simulink model "model"  (R2024b)
settings: Solver=VariableStepAuto  StartTime=0.0  StopTime=10.0  RelTol=1e-3
undefined symbols (not defined in the file): k
libraries: arduinolib x3, simulink_extras x2, eeGeneralControl x2
settings Model: Creator=eslam  LastModifiedBy=eslam

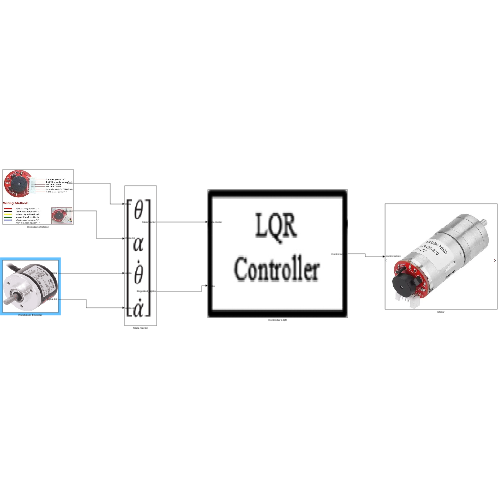
[thumbnail: Simulink's stored preview of the top-level diagram]
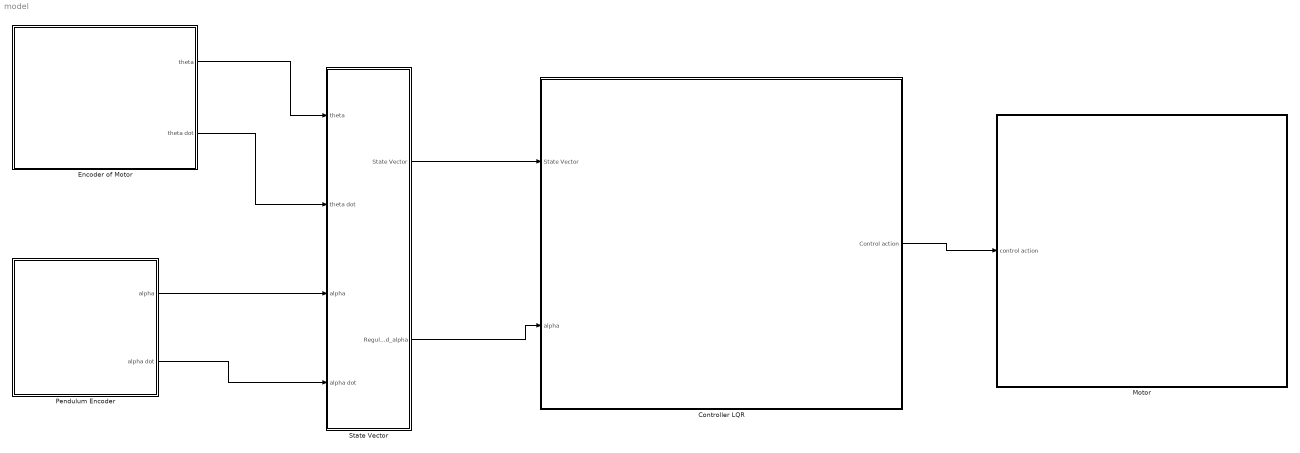
== system model ==
  Controller LQR : Subsystem
      mask Display: image('lqr.PNG');
  Encoder of Motor : Subsystem
      mask Display: image('Motor Encoder.jpeg');
  Motor : Subsystem
      mask Display: image('Motor.png');
  Pendulum Encoder : Subsystem
      mask Display: image('Encoder.png');
  State Vector : Subsystem
      mask Display: image('States.PNG');
  wires:
  Encoder of Motor/1(theta) -> State Vector/1(theta)
  Pendulum Encoder/1(alpha) -> State Vector/3(alpha)
  Encoder of Motor/2(theta dot) -> State Vector/2(theta dot)
  Pendulum Encoder/2(alpha dot) -> State Vector/4(alpha dot)
  State Vector/1(State Vector) -> Controller LQR/1(State Vector)
  State Vector/2(Regulated_alpha) -> Controller LQR/2(alpha)
  Controller LQR/1(Control action) -> Motor/1("control action ")

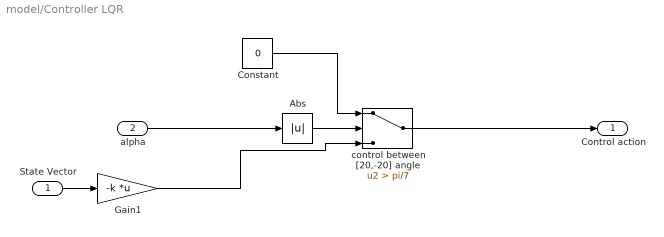
== system model/Controller LQR ==
  State Vector : Inport
  alpha : Inport  Port=2
  Abs : Abs  SaturateOnIntegerOverflow=off
  Constant : Constant  Value=0
  Gain1 : Gain  Gain=-k  Multiplication=Matrix(K*u)
  control between [20,-20] angle : Switch  Criteria=u2 > Threshold  Threshold=pi/7  SaturateOnIntegerOverflow=off  InputSameDT=off
  Control action : Outport
  wires:
  Abs/1 -> control between [20,-20] angle/2
  control between [20,-20] angle/1 -> Control action/1
  alpha/1 -> Abs/1
  Constant/1 -> control between [20,-20] angle/1
  State Vector/1 -> Gain1/1
  Gain1/1 -> control between [20,-20] angle/3

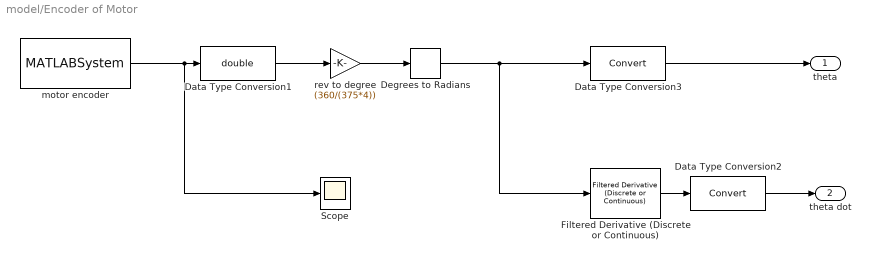
== system model/Encoder of Motor ==
  Data Type Conversion1 : DataTypeConversion  OutDataTypeStr=double  SaturateOnIntegerOverflow=off  RndMeth=Floor
  Data Type Conversion2 : DataTypeConversion  SaturateOnIntegerOverflow=off  RndMeth=Floor
  Data Type Conversion3 : DataTypeConversion  SaturateOnIntegerOverflow=off  RndMeth=Floor
  Degrees to Radians : simulink_extras/Transformations/Degrees to Radians
  Filtered Derivative (Discrete or Continuous) : eeGeneralControl/Filtered Derivative (Discrete or Continuous)  K=-1  T=0.001  B=inf  A=-inf  minRatio=10  init_option=Inherited from block input  x0=0  Ts=-1
  Scope : Scope
  motor encoder : MATLABSystem  System=Encoder_arduino  Encoder=1  PinA=3  PinB=5  SampleTime=0.001
  rev to degree : Gain  Gain=(360/(375*4))
  theta : Outport
  theta dot : Outport  Port=2
  wires:
  motor encoder/1 -> Scope/1, Data Type Conversion1/1
  Degrees to Radians/1 -> Filtered Derivative (Discrete or Continuous)/1, Data Type Conversion3/1
  Data Type Conversion3/1 -> theta/1
  Data Type Conversion2/1 -> theta dot/1
  Data Type Conversion1/1 -> rev to degree/1
  rev to degree/1 -> Degrees to Radians/1
  Filtered Derivative (Discrete or Continuous)/1 -> Data Type Conversion2/1

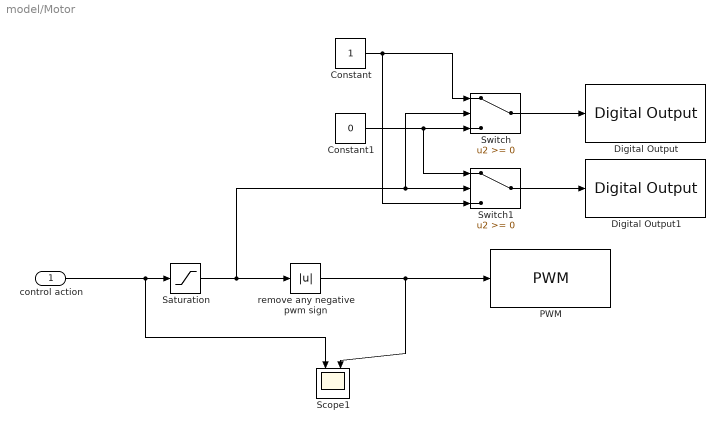
== system model/Motor ==
  "control action " : Inport
  Constant : Constant
  Constant1 : Constant  Value=0
  Digital Output : arduinolib/Digital Output  pinNumber=9  Direction=output  blockPlatform=arduino
  Digital Output1 : arduinolib/Digital Output  pinNumber=8  Direction=output  blockPlatform=arduino
  PWM : arduinolib/PWM  pinNumber=6  frequencyType=Default  desiredFrequency=490.2  achievableFrequency=490.2
  Saturation : Saturate  UpperLimit=255  LowerLimit=-255
  Scope1 : Scope  NumInputPorts=2
  Switch : Switch  SaturateOnIntegerOverflow=off  InputSameDT=off
  Switch1 : Switch  SaturateOnIntegerOverflow=off  InputSameDT=off
  remove any negative pwm sign : Abs  SaturateOnIntegerOverflow=off
  wires:
  "control action "/1 -> Scope1/1, Saturation/1
  Constant/1 -> Switch/1, Switch1/3
  Switch/1 -> Digital Output/1
  Constant1/1 -> Switch1/1, Switch/3
  remove any negative pwm sign/1 -> Scope1/2, PWM/1
  Switch1/1 -> Digital Output1/1
  Saturation/1 -> Switch/2, Switch1/2, remove any negative pwm sign/1

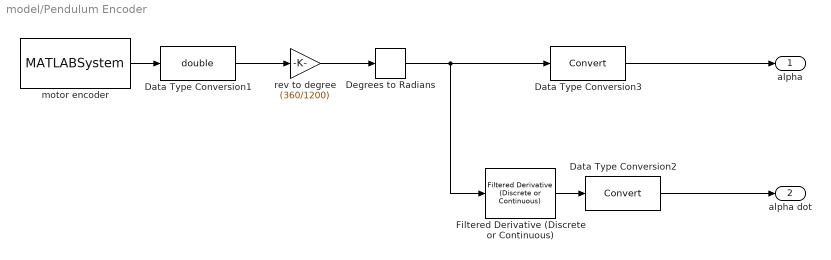
== system model/Pendulum Encoder ==
  Data Type Conversion1 : DataTypeConversion  OutDataTypeStr=double  SaturateOnIntegerOverflow=off  RndMeth=Floor
  Data Type Conversion2 : DataTypeConversion  SaturateOnIntegerOverflow=off  RndMeth=Floor
  Data Type Conversion3 : DataTypeConversion  SaturateOnIntegerOverflow=off  RndMeth=Floor
  Degrees to Radians : simulink_extras/Transformations/Degrees to Radians
  Filtered Derivative (Discrete or Continuous) : eeGeneralControl/Filtered Derivative (Discrete or Continuous)  K=1  T=0.001  B=inf  A=-inf  minRatio=10  init_option=Inherited from block input  x0=0  Ts=-1
  motor encoder : MATLABSystem  System=Encoder_arduino  Encoder=0  PinA=2  PinB=4  SampleTime=0.001
  rev to degree : Gain  Gain=(360/1200)
  alpha : Outport
  alpha dot : Outport  Port=2
  wires:
  Filtered Derivative (Discrete or Continuous)/1 -> Data Type Conversion2/1
  Data Type Conversion2/1 -> alpha dot/1
  Data Type Conversion3/1 -> alpha/1
  Data Type Conversion1/1 -> rev to degree/1
  Degrees to Radians/1 -> Filtered Derivative (Discrete or Continuous)/1, Data Type Conversion3/1
  motor encoder/1 -> Data Type Conversion1/1
  rev to degree/1 -> Degrees to Radians/1

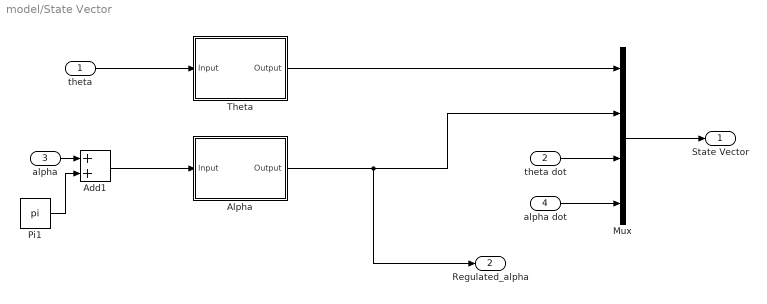
== system model/State Vector ==
  theta : Inport
  theta dot : Inport  Port=2
  alpha : Inport  Port=3
  alpha dot : Inport  Port=4
  Add1 : Sum
  Alpha : Subsystem
  Mux : Mux
  Pi1 : Constant  Value=pi  OutDataTypeStr=Inherit: Inherit via back propagation
  Theta : Subsystem
  State Vector : Outport
  Regulated_alpha : Outport  Port=2
  wires:
  theta/1 -> Theta/1(Input)
  Add1/1 -> Alpha/1(Input)
  alpha/1 -> Add1/1
  Pi1/1 -> Add1/2
  Mux/1 -> State Vector/1
  Theta/1(Output) -> Mux/1
  Alpha/1(Output) -> Regulated_alpha/1, Mux/2
  theta dot/1 -> Mux/3
  alpha dot/1 -> Mux/4

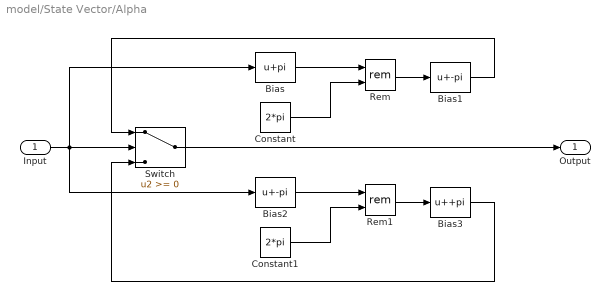
== system model/State Vector/Alpha ==
  Input : Inport
  Bias : Bias  Bias=pi  SaturateOnIntegerOverflow=off
  Bias1 : Bias  Bias=-pi  SaturateOnIntegerOverflow=off
  Bias2 : Bias  Bias=-pi  SaturateOnIntegerOverflow=off
  Bias3 : Bias  Bias=+pi  SaturateOnIntegerOverflow=off
  Constant : Constant  Value=2*pi
  Constant1 : Constant  Value=2*pi
  Rem : Math  Operator=rem
  Rem1 : Math  Operator=rem
  Switch : Switch  SaturateOnIntegerOverflow=off  InputSameDT=off
  Output : Outport
  wires:
  Bias1/1 -> Switch/1
  Rem/1 -> Bias1/1
  Switch/1 -> Output/1
  Constant1/1 -> Rem1/2
  Rem1/1 -> Bias3/1
  Bias2/1 -> Rem1/1
  Bias3/1 -> Switch/3
  Input/1 -> Switch/2, Bias2/1, Bias/1
  Bias/1 -> Rem/1
  Constant/1 -> Rem/2

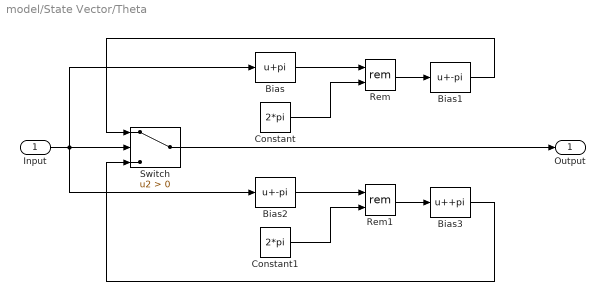
== system model/State Vector/Theta ==
  Input : Inport
  Bias : Bias  Bias=pi  SaturateOnIntegerOverflow=off
  Bias1 : Bias  Bias=-pi  SaturateOnIntegerOverflow=off
  Bias2 : Bias  Bias=-pi  SaturateOnIntegerOverflow=off
  Bias3 : Bias  Bias=+pi  SaturateOnIntegerOverflow=off
  Constant : Constant  Value=2*pi
  Constant1 : Constant  Value=2*pi
  Rem : Math  Operator=rem
  Rem1 : Math  Operator=rem
  Switch : Switch  Criteria=u2 > Threshold  SaturateOnIntegerOverflow=off  InputSameDT=off
  Output : Outport
  wires:
  Constant/1 -> Rem/2
  Bias/1 -> Rem/1
  Input/1 -> Bias/1, Bias2/1, Switch/2
  Bias3/1 -> Switch/3
  Bias2/1 -> Rem1/1
  Rem1/1 -> Bias3/1
  Constant1/1 -> Rem1/2
  Switch/1 -> Output/1
  Rem/1 -> Bias1/1
  Bias1/1 -> Switch/1
